simulink model "Fig345"  (R2014b)
settings: Solver=ode3  StartTime=0.0  StopTime=10.002  FixedStep=2e-6  RelTol=1e-5
libraries: commfilt2 x1, commchan3 x1, commsink2 x1, dsparch4 x1, commanapbnd3 x1, commrandsrc2 x1
settings Model: Creator=Dennis Silage  LastModifiedBy=Silage
settings DataIOCC: SignalLoggingSaveFormat=ModelDataLogs
settings OptimizationCC: ExpressionDepthLimit=2147483647  InitFltsAndDblsToZero=on
settings DebuggingCC: UnderspecifiedInitializationDetection=Classic  MergeDetectMultiDrivingBlocksExec=none  SolverPrmCheckMsg=none  FcnCallInpInsideContextMsg=UseLocalSettings  StateNameClashWarn=warning
settings GRTTargetCC: CombineOutputUpdateFcns=off  GRTInterface=on

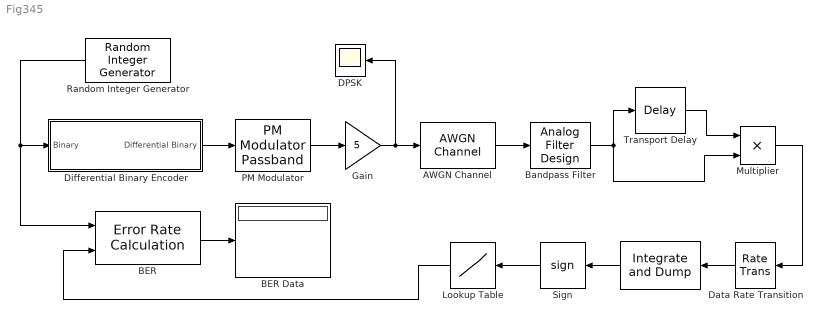
== system Fig345 ==
  " " : commfilt2/Integrate and Dump  obssamples=500  offsetsamples=0  nodump=off  roundingMode=Floor  overflowMode=off
  AWGN Channel : commchan3/AWGN Channel  InputProcessing=Inherited (this choice will be removed - see release notes)  seed=randseed  noiseMode="Signal to noise ratio  (Eb/No)"  EbNodB=50  EsNodB=10  SNRdB=12  bitsPerSym=1  Ps=12.5  Tsym=1e-3  variance=0
  BER : commsink2/Error Rate Calculation  N=3  st_delay=0  cp_mode=Entire frame  subframe=[]  PMode=Port  WsName=ErrorVec  RsMode2=off  stop=off  numErr=100  maxBits=1e6
  BER Data : Display
  Bandpass Filter : dsparch4/Analog Filter Design  method=Butterworth  filttype=Bandpass  N=9  Wlo=38000*pi  Whi=42000*pi  Rp=2  Rs=40
  DPSK : Scope
      settings: YMin=-6  YMax=6
  Data Rate Transition : RateTransition  OutPortSampleTime=2e-6
  Differential Binary Encoder : Subsystem
  Gain : Gain  Gain=5
  Lookup Table : Lookup_n-D  NumberOfTableDimensions=1  BreakpointsForDimension1=[-1,0,1]  Table=[0,0,1]  InternalRulePriority=Speed  RndMeth=Simplest  InputSameDT=on
  Multiplier : Product  RndMeth=Zero
  PM Modulator : commanapbnd3/PM Modulator Passband  Fc=20000  Ph=pi  Kc=pi
  Random Integer Generator : commrandsrc2/Random Integer Generator  mul=2  seed=randseed  Ts=1e-3  frameBased=off  sampPerFrame=50  orient=on  outDataType=double
  Sign : Signum
  Transport Delay : TransportDelay  DelayTime=.001
  wires:
  BER/1 -> BER Data/1
  Gain/1 -> AWGN Channel/1, DPSK/1
  PM Modulator/1 -> Gain/1
  AWGN Channel/1 -> Bandpass Filter/1
  Bandpass Filter/1 -> Multiplier/2, Transport Delay/1
  Differential Binary Encoder/1(Differential Binary) -> PM Modulator/1
  Random Integer Generator/1 -> Differential Binary Encoder/1(Binary), BER/1
  " "/1 -> Sign/1
  Multiplier/1 -> Data Rate Transition/1
  Data Rate Transition/1 -> " "/1
  Transport Delay/1 -> Multiplier/1
  Sign/1 -> Lookup Table/1
  Lookup Table/1 -> BER/2

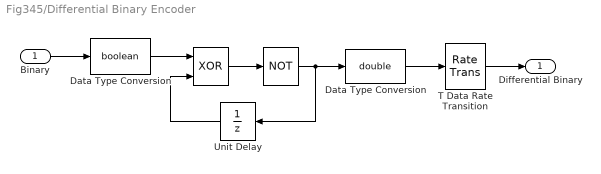
== system Fig345/Differential Binary Encoder ==
  Binary : Inport
  " " : Logic  Operator=NOT  IconShape=distinctive
  "  " : Logic  Operator=XOR  IconShape=distinctive
  Data Type Conversion : DataTypeConversion  OutDataTypeStr=double
  "Data Type Conversion " : DataTypeConversion  OutDataTypeStr=boolean
  T Data Rate Transition : RateTransition  OutPortSampleTime=2e-6
  Unit Delay : UnitDelay  SampleTime=-1
  Differential Binary : Outport
  wires:
  Unit Delay/1 -> "  "/2
  Data Type Conversion/1 -> T Data Rate Transition/1
  "  "/1 -> " "/1
  T Data Rate Transition/1 -> Differential Binary/1
  " "/1 -> Data Type Conversion/1, Unit Delay/1
  "Data Type Conversion "/1 -> "  "/1
  Binary/1 -> "Data Type Conversion "/1
